simulink model "CLAPAR"  (R2022b)
settings: configuration reference "SharedConfig" (kept outside this file)
values from neighbouring files (symbols this model uses):
  PhaCurDDialEna_C = 0.0    [CLAPAR.sldd]
  PhaCurDDialVal_C = 0.0    [CLAPAR.sldd]
  PhaCurQDialEna_C = 0.0    [CLAPAR.sldd]
  PhaCurQDialVal_C = 0.0    [CLAPAR.sldd]
undefined symbols (not defined in the file or in its folder): slcm
Description:
  | Converts the phase currents in the abc phase reference frame into the dq rotating reference frame.
settings Model: DataDictionary=CLAPAR.sldd  Creator=Kevin  LastModifiedBy=Max Kolesnikov
settings ConfigSetRef: SourceName=SharedConfig

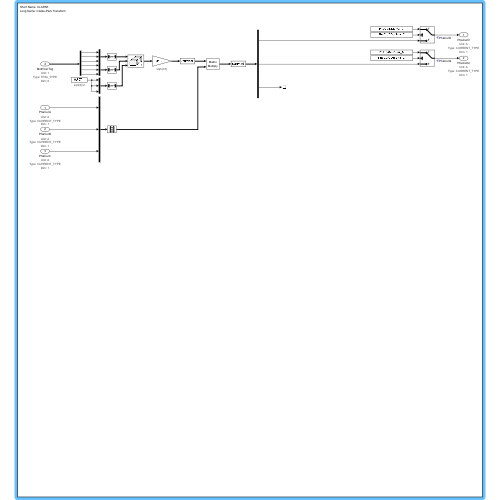
[thumbnail: Simulink's stored preview of the top-level diagram]
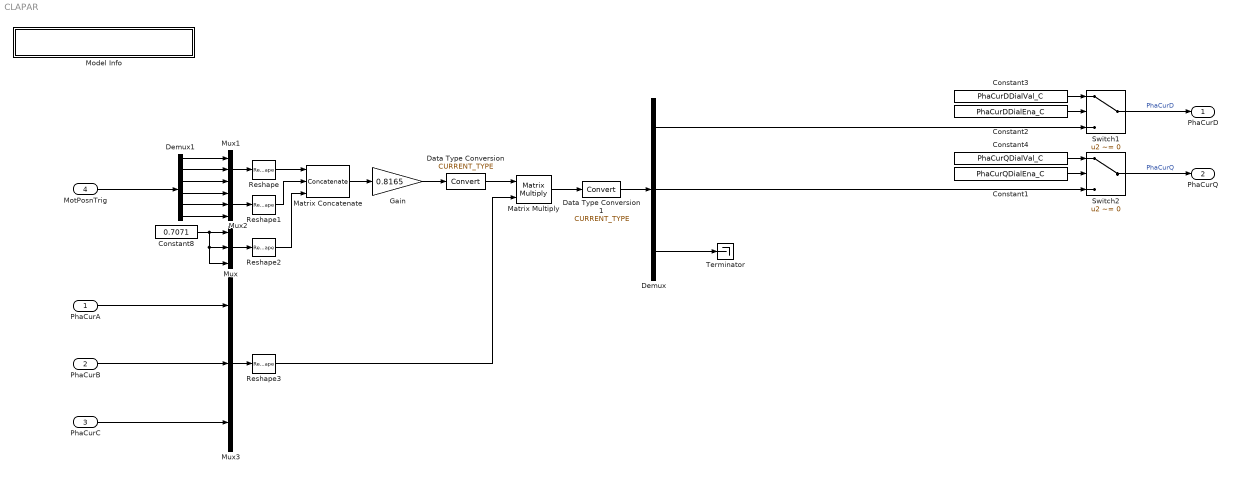
== system CLAPAR ==
  PhaCurA : Inport  OutDataTypeStr=CURRENT_TYPE  Unit=A  PortDimensions=1
      settings: AttributesFormatString=|
      | Unit: %<Unit>
      | Type: %<OutDataTypeStr>
      | Dim: %<PortDimensions>
  PhaCurB : Inport  Port=2  OutDataTypeStr=CURRENT_TYPE  Unit=A  PortDimensions=1
      settings: AttributesFormatString=|
      | Unit: %<Unit>
      | Type: %<OutDataTypeStr>
      | Dim: %<PortDimensions>
  PhaCurC : Inport  Port=3  OutDataTypeStr=CURRENT_TYPE  Unit=A  PortDimensions=1
      settings: AttributesFormatString=|
      | Unit: %<Unit>
      | Type: %<OutDataTypeStr>
      | Dim: %<PortDimensions>
  MotPosnTrig : Inport  Port=4  OutDataTypeStr=TRIG_TYPE  Unit=1  PortDimensions=6
      settings: AttributesFormatString=|
      | Unit: %<Unit>
      | Type: %<OutDataTypeStr>
      | Dim: %<PortDimensions>
  Constant1 : Constant  Value=PhaCurQDialEna_C
  Constant2 : Constant  Value=PhaCurDDialEna_C
  Constant3 : Constant  Value=PhaCurDDialVal_C
  Constant4 : Constant  Value=PhaCurQDialVal_C
  Constant8 : Constant  Description=sqrt(2)/2  Value=0.7071  OutDataTypeStr=TRIG_TYPE
      settings: AttributesFormatString=%<Description>
  Data Type Conversion : DataTypeConversion  OutDataTypeStr=CURRENT_TYPE  SaturateOnIntegerOverflow=off  RndMeth=Floor
  Data Type Conversion1 : DataTypeConversion  OutDataTypeStr=CURRENT_TYPE  SaturateOnIntegerOverflow=off  RndMeth=Floor
  Demux : Demux  Outputs=3
  Demux1 : Demux  Outputs=6
  Gain : Gain  Description=sqrt(2/3)  Gain=0.8165
      settings: AttributesFormatString=%<Description>
  Matrix Concatenate : Concatenate  NumInputs=3  Mode=Multidimensional array
  Matrix Multiply : Product  Multiplication=Matrix(*)
  Model Info : Subsystem  LoadFcn=slcm LoadBlock;  InitFcn=slcm('UpdateAllCMBlocksInThisModelInit')  mask(CMBlock){Frame=off, DisplayStringWithTags=|, MaskDisplayString=Short Name: CLAPAR\nLong Name: Clarke-Park Transform, HorizontalTextAlignment=Left, LeftAlignmentValue=0.02}
      mask DisplayStringWithTags=|
      | Short Name: %<ModelName>
      | Long Name: Clarke-Park Transform
      mask prompts: Frame "Simulink:masks:Frame_MP"; DisplayStringWithTags "Simulink:masks:DisplayStringWithTags_MP"; MaskDisplayString "Simulink:masks:MaskDisplayString_MP"; HorizontalTextAlignment "Simulink:masks:HorizontalTextAlignment_MP"; LeftAlignmentValue "Simulink:masks:LeftAlignmentValue_MP"
      mask help: Simulink:masks:CMBlock_MD
      settings: CopyFcn=slcm CopyBlock;  DeleteFcn=slcm Cancel;  PostSaveFcn=slcm('UpdateAllCMBlocksInThisModel')  NameChangeFcn=slcm Rename;  OpenFcn=slcm
      mask Display: text(slResolve(LeftAlignmentValue, gcbh), 0.5, MaskDisplayString, 'HorizontalAlignment', HorizontalTextAlignment)
  Mux{,1..3} (4 alike) : Mux  Inputs=3
  Reshape : Reshape  OutputDimensionality=Row vector (2-D)
  Reshape1 : Reshape  OutputDimensionality=Row vector (2-D)
  Reshape2 : Reshape  OutputDimensionality=Row vector (2-D)
  Reshape3 : Reshape  OutputDimensionality=Column vector (2-D)
  Switch1 : Switch  Criteria=u2 ~= 0  SaturateOnIntegerOverflow=off  InputSameDT=off
  Switch2 : Switch  Criteria=u2 ~= 0  SaturateOnIntegerOverflow=off  InputSameDT=off
  Terminator : Terminator
  PhaCurD : Outport  OutDataTypeStr=CURRENT_TYPE  Unit=A  PortDimensions=1
      settings: AttributesFormatString=|
      | Unit: %<Unit>
      | Type: %<OutDataTypeStr>
      | Dim: %<PortDimensions>
  PhaCurQ : Outport  Port=2  OutDataTypeStr=CURRENT_TYPE  Unit=A  PortDimensions=1
      settings: AttributesFormatString=|
      | Unit: %<Unit>
      | Type: %<OutDataTypeStr>
      | Dim: %<PortDimensions>
  wires:
  Constant3/1 -> Switch1/1
  Constant2/1 -> Switch1/2
  Switch1/1 -> PhaCurD/1  "PhaCurD"
  Switch2/1 -> PhaCurQ/1  "PhaCurQ"
  Constant1/1 -> Switch2/2
  Constant4/1 -> Switch2/1
  Constant8/1 -> Mux/3, Mux/2, Mux/1
  Mux/1 -> Reshape2/1
  Matrix Concatenate/1 -> Gain/1
  PhaCurA/1 -> Mux3/1
  PhaCurB/1 -> Mux3/2
  PhaCurC/1 -> Mux3/3
  Gain/1 -> Data Type Conversion/1
  Mux3/1 -> Reshape3/1
  Matrix Multiply/1 -> Data Type Conversion1/1
  Demux/1 -> Switch1/3
  Demux/2 -> Switch2/3
  Demux/3 -> Terminator/1
  MotPosnTrig/1 -> Demux1/1
  Demux1/1 -> Mux1/1
  Demux1/2 -> Mux1/2
  Demux1/3 -> Mux1/3
  Demux1/4 -> Mux2/1
  Demux1/5 -> Mux2/2
  Demux1/6 -> Mux2/3
  Mux1/1 -> Reshape/1
  Mux2/1 -> Reshape1/1
  Reshape/1 -> Matrix Concatenate/1
  Reshape1/1 -> Matrix Concatenate/2
  Reshape2/1 -> Matrix Concatenate/3
  Reshape3/1 -> Matrix Multiply/2
  Data Type Conversion/1 -> Matrix Multiply/1
  Data Type Conversion1/1 -> Demux/1

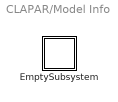
== system CLAPAR/Model Info ==
  EmptySubsystem : Subsystem

== system CLAPAR/Model Info/EmptySubsystem ==
